simulink model "parallelss"  (Simulink 8.1)
settings: Solver=ode45  StartTime=0.0  StopTime=10.0  RelTol=1e-3
values from neighbouring files (symbols this model uses):
  x1 = (A-B*K)*x0    [optimiser_setup.m]
undefined symbols (not defined in the file or in its folder): A1, A2
libraries: Is_equal_scalar x1, goal x1
settings Model: Creator=dejanira  LastModifiedBy=dejanira
settings DataIOCC: SignalLoggingSaveFormat=Dataset
settings OptimizationCC: ExpressionDepthLimit=128
settings DebuggingCC: FcnCallInpInsideContextMsg=EnableAllAsError
settings GRTTargetCC: CombineOutputUpdateFcns=on  GRTInterface=off

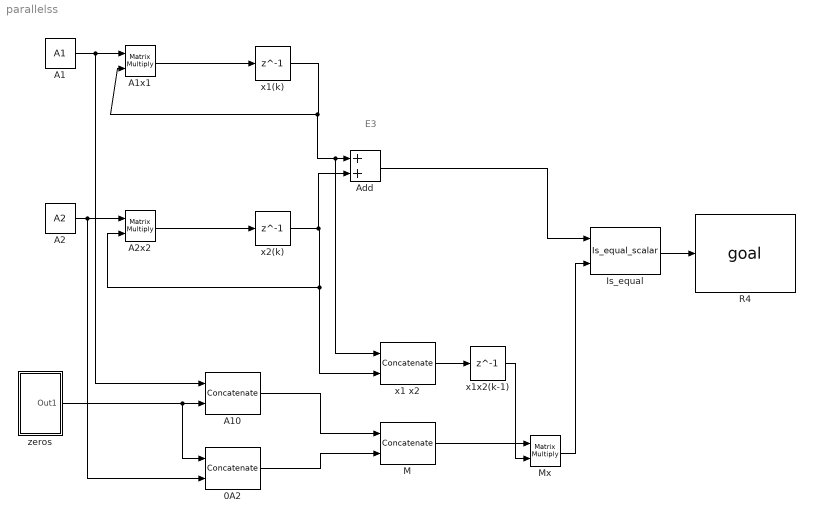
== system parallelss ==
  note: E3
  0A2 : Concatenate  Mode=Multidimensional array  ConcatenateDimension=2
  A1 : Constant  Value=A1  VectorParams1D=off
  A10 : Concatenate  Mode=Multidimensional array  ConcatenateDimension=2
  A1x1 : Product  Multiplication=Matrix(*)
  A2 : Constant  Value=A2  VectorParams1D=off
  A2x2 : Product  Multiplication=Matrix(*)
  Add : Sum
  Is_equal : Is_equal_scalar/Is_equal_scalar  SystemSampleTime=-1
  M : Concatenate  Mode=Multidimensional array
  Mx : Product  Multiplication=Matrix(*)
  R4 : goal/goal  SystemSampleTime=-1
  x1 x2 : Concatenate  Mode=Multidimensional array
  x1(k) : Delay  DelayLength=1  InitialCondition=x1  SampleTime=0.1
  x1x2(k-1) : Delay  DelayLength=1  InitialCondition=x1  SampleTime=0.1
  x2(k) : Delay  DelayLength=1  InitialCondition=x1  SampleTime=0.1
  zeros : Subsystem  mask(m0){}
  wires:
  x1(k)/1 -> x1 x2/1, Add/1, A1x1/2
  A1/1 -> A10/1, A1x1/1
  x2(k)/1 -> Add/2, x1 x2/2, A2x2/2
  A2x2/1 -> x2(k)/1
  A1x1/1 -> x1(k)/1
  x1 x2/1 -> x1x2(k-1)/1
  M/1 -> Mx/1
  x1x2(k-1)/1 -> Mx/2
  zeros/1(Out1) -> 0A2/1, A10/2
  A10/1 -> M/1
  0A2/1 -> M/2
  A2/1 -> 0A2/2, A2x2/1
  Add/1 -> Is_equal/1
  Is_equal/1 -> R4/1
  Mx/1 -> Is_equal/2

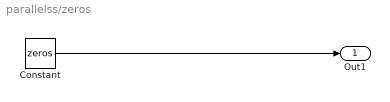
== system parallelss/zeros ==
  Constant : Constant  Value=zeros  VectorParams1D=off
  Out1 : Outport
  wires:
  Constant/1 -> Out1/1
